simulink model "rendszer"  (R2020b)
settings: Solver=ode45  StartTime=0.0  StopTime=50  MaxStep=1e-3  RelTol=1e-3
settings Model: Creator=Legion1  LastModifiedBy=Legion1

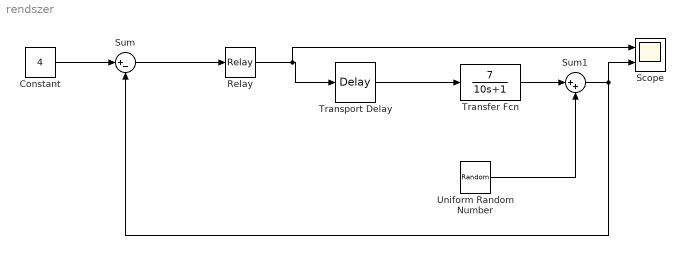
== system rendszer ==
  Constant : Constant  Value=4
  Relay : Relay  OnSwitchValue=0.1  OffSwitchValue=-0.1
  Scope : Scope  NumInputPorts=2
  Sum : Sum  Inputs=|+-
  Sum1 : Sum  Inputs=|++
  Transfer Fcn : TransferFcn  Numerator=[7]  Denominator=[10 1]
  Transport Delay : TransportDelay  DelayTime=3
  Uniform Random Number : UniformRandomNumber  Minimum=-0.1  Maximum=0.1  SampleTime=0.1
  wires:
  Transport Delay/1 -> Transfer Fcn/1
  Constant/1 -> Sum/1
  Transfer Fcn/1 -> Sum1/1
  Sum1/1 -> Scope/2, Sum/2
  Uniform Random Number/1 -> Sum1/2
  Relay/1 -> Scope/1, Transport Delay/1
  Sum/1 -> Relay/1
